simulink model "model_3D_Lissajous"  (R2020b)
settings: Solver=ode4  StartTime=0.0  StopTime=20  FixedStep=0.01  RelTol=1e-3
settings Model: Creator=70952  LastModifiedBy=70952

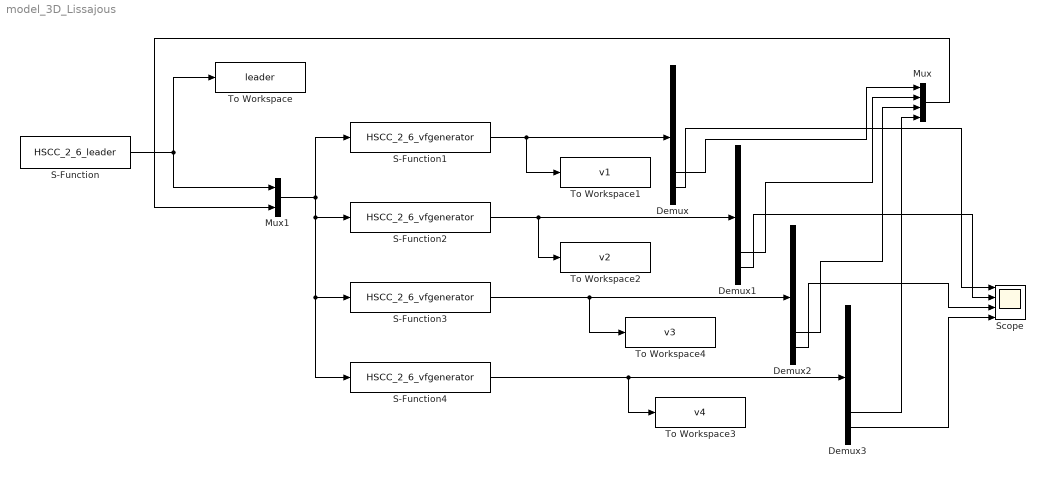
== system model_3D_Lissajous ==
  Demux{,1..3} (4 alike) : Demux  Outputs=8
  Mux : Mux
  Mux1 : Mux  Inputs=2
  S-Function : S-Function  FunctionName=HSCC_2_6_leader  SFunctionDeploymentMode=off  EnableBusSupport=off
  S-Function1 : S-Function  FunctionName=HSCC_2_6_vfgenerator  Parameters=[1 0 0 0],1  SFunctionDeploymentMode=off  EnableBusSupport=off
  S-Function2 : S-Function  FunctionName=HSCC_2_6_vfgenerator  Parameters=[1 1 0 0],2  SFunctionDeploymentMode=off  EnableBusSupport=off
  S-Function3 : S-Function  FunctionName=HSCC_2_6_vfgenerator  Parameters=[-1 0 0 0],3  SFunctionDeploymentMode=off  EnableBusSupport=off
  S-Function4 : S-Function  FunctionName=HSCC_2_6_vfgenerator  Parameters=[1 0 2 0],4  SFunctionDeploymentMode=off  EnableBusSupport=off
  Scope : Scope  NumInputPorts=4
  To Workspace : ToWorkspace  VariableName=leader  SampleTime=-1
  To Workspace1 : ToWorkspace  VariableName=v1  SampleTime=-1
  To Workspace2 : ToWorkspace  VariableName=v2  SampleTime=-1
  To Workspace3 : ToWorkspace  VariableName=v4  SampleTime=-1
  To Workspace4 : ToWorkspace  VariableName=v3  SampleTime=-1
  wires:
  S-Function/1 -> To Workspace/1, Mux1/1
  S-Function1/1 -> Demux/1, To Workspace1/1
  S-Function2/1 -> To Workspace2/1, Demux1/1
  S-Function4/1 -> To Workspace3/1, Demux3/1
  S-Function3/1 -> To Workspace4/1, Demux2/1
  Demux/7 -> Mux/1
  Demux1/7 -> Mux/2
  Demux2/7 -> Mux/3
  Demux3/7 -> Mux/4
  Mux/1 -> Mux1/2
  Mux1/1 -> S-Function1/1, S-Function4/1, S-Function3/1, S-Function2/1
  Demux/8 -> Scope/1
  Demux1/8 -> Scope/2
  Demux2/8 -> Scope/3
  Demux3/8 -> Scope/4
